simulink model "tp1_feedback"  (R2023a)
settings: Solver=VariableStepAuto  StartTime=0.0  StopTime=10.0  RelTol=1e-3
values from neighbouring files (symbols this model uses):
  A = [0 1 0 0 ; ((M+m)*g)/(M*L) 0 0 0; 0 0 0 1; (-m*g)/M 0 0 0]    [TP1.m]
  B = [0; -1/M*L;0;1/M]    [TP1.m]
  C_block = eye(4)    [TP1.m]
  D = [0;0;0;0]    [TP1.m]
  F = -place(A,B,p_desired)    [TP1.m]
  x_0 = [0.1;0;0.1;0]    [TP1.m]
settings Model: Creator=jlancha2023  LastModifiedBy=jlancha2023

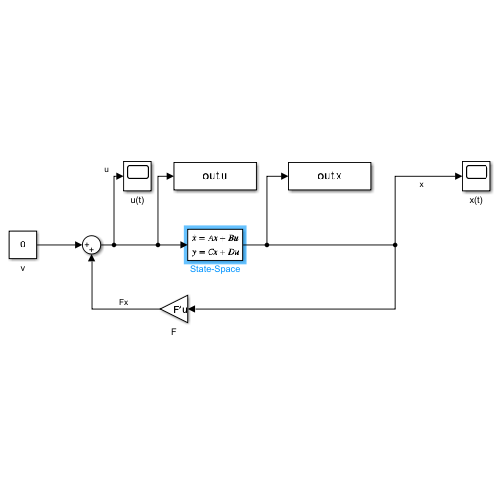
[thumbnail: Simulink's stored preview of the top-level diagram]
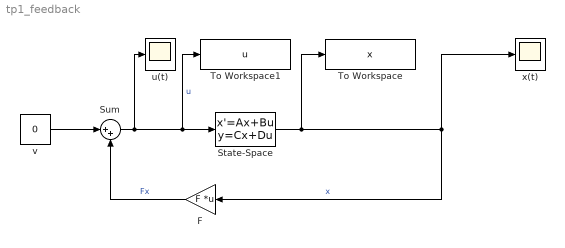
== system tp1_feedback ==
  F : Gain  Gain=F  Multiplication=Matrix(K*u)
  State-Space : StateSpace  A=A  B=B  C=C_block  D=D  InitialCondition=x_0
  Sum : Sum  Inputs=|++
  To Workspace : ToWorkspace  VariableName=x  SampleTime=-1
  To Workspace1 : ToWorkspace  VariableName=u  SampleTime=-1
  u(t) : Scope
  v : Constant  Value=0
  x(t) : Scope
  wires:
  Sum/1 -> u(t)/1, To Workspace1/1, State-Space/1  "u"
  State-Space/1 -> F/1, x(t)/1, To Workspace/1  "x"
  F/1 -> Sum/2  "Fx"
  v/1 -> Sum/1
